simulink model "dynamics"  (R2024a)
settings: Solver=VariableStepAuto  StartTime=0.0  StopTime=10.0  RelTol=1e-3
undefined symbols (not defined in the file): Angle_init, Omega_init, V_init
settings Model: Creator=10335  LastModifiedBy=10335

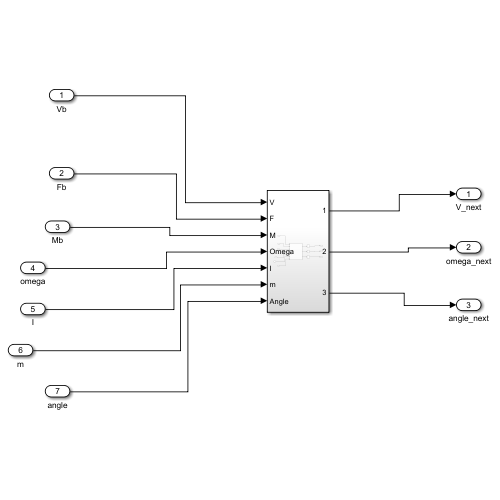
[thumbnail: Simulink's stored preview of the top-level diagram]
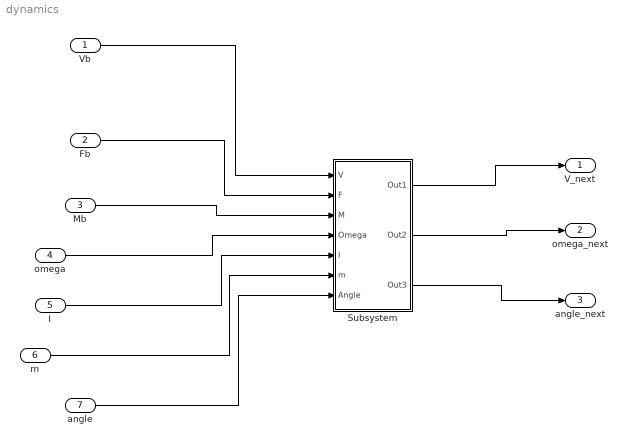
== system dynamics ==
  Vb : Inport
  Fb : Inport  Port=2
  Mb : Inport  Port=3
  omega : Inport  Port=4
  I : Inport  Port=5
  m : Inport  Port=6
  angle : Inport  Port=7
  Subsystem : Subsystem
  V_next : Outport
  omega_next : Outport  Port=2
  angle_next : Outport  Port=3
  wires:
  Vb/1 -> Subsystem/1(V)
  Fb/1 -> Subsystem/2(F)
  Mb/1 -> Subsystem/3(M)
  omega/1 -> Subsystem/4(Omega)
  I/1 -> Subsystem/5(I)
  m/1 -> Subsystem/6(m)
  angle/1 -> Subsystem/7(Angle)
  Subsystem/1(Out1) -> V_next/1
  Subsystem/2(Out2) -> omega_next/1
  Subsystem/3(Out3) -> angle_next/1

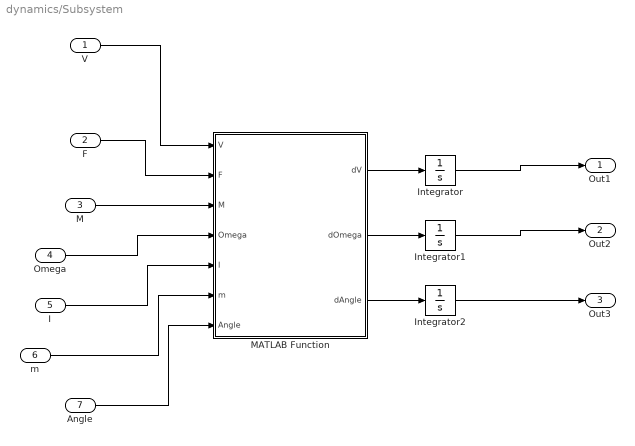
== system dynamics/Subsystem ==
  V : Inport
  F : Inport  Port=2
  M : Inport  Port=3
  Omega : Inport  Port=4
  I : Inport  Port=5
  m : Inport  Port=6
  Angle : Inport  Port=7
  Integrator : Integrator  InitialCondition=V_init
  Integrator1 : Integrator  InitialCondition=Omega_init
  Integrator2 : Integrator  InitialCondition=Angle_init
  MATLAB Function : MATLAB Function  TreatAsAtomicUnit=on
  Out1 : Outport
  Out2 : Outport  Port=2
  Out3 : Outport  Port=3
  wires:
  Omega/1 -> MATLAB Function/4(Omega)
  m/1 -> MATLAB Function/6(m)
  MATLAB Function/1(dV) -> Integrator/1
  Integrator1/1 -> Out2/1
  MATLAB Function/3(dAngle) -> Integrator2/1
  I/1 -> MATLAB Function/5(I)
  Integrator/1 -> Out1/1
  F/1 -> MATLAB Function/2(F)
  MATLAB Function/2(dOmega) -> Integrator1/1
  M/1 -> MATLAB Function/3(M)
  Integrator2/1 -> Out3/1
  Angle/1 -> MATLAB Function/7(Angle)
  V/1 -> MATLAB Function/1(V)

== matlab function dynamics/Subsystem/MATLAB Function ==
  data: V input; dV output; F input; M input; Omega input; I input; m input; Angle input; dOmega output; dAngle output
function [dV,dOmega,dAngle] = fcn(V,F,M,Omega,I,m,Angle)

Vx=V(1);
Vy=V(2);
Vz=V(3);

Fx=F(1);
Fy=F(2);
Fz=F(3);

Mx=M(1);
My=M(2);
Mz=M(3);

Wx=Omega(1);
Wy=Omega(2);
Wz=Omega(3);

theta=Angle(1);
phi=Angle(2);
rama=Angle(3);

Ixx=I(1,1);
Iyy=I(2,2);
Izz=I(3,3);
Ixy=I(1,2);


dVx=Fx/m-g*sin(theta)-(Vz*Wy-Vy*Wz);
dVy=Fy/m-g*cos(theta)*cos(rama)-(Vx*Wz-Vz*Wx);
dVz=Fz/m+g*cos(theta)*sin(rama)-(Vy*Wx-Vx*Wy);

dWz=(Mz-Ixy*(Wy*Wy-Wx*Wx)-Wx*Wy(Iyy-Ixx))/Izz;

A=Mx-Wy*Wz*(Izz-Iyy);
B=My-Wx*Wz*(Ixx-Izz);
dWx=(A+Ixy*B/Iyy)/(Ixx+Ixy*Ixy/Iyy);
dWy=(B-Ixy*A/Ixx)/(Iyy+Ixy*Ixy/Ixx);


dtheta=Wz*cos(rama)+Wy*sin(rama);
drama=Wx-tan(theta)*(Wy*cos(rama)-Wz*sin(rama));
dphi=(Wy*cos(rama)-Wz*sin(rama))/cos(theta);


dV=[dVx,dVy,dVz]';
dOmega=[dWx,dWy,dWz];
dAngle=[dtheta,dphi,drama]';
